simulink model "Current_Controller"  (Simulink 8.9)
settings: Solver=VariableStepAuto  StartTime=0.0  StopTime=0.5  RelTol=1e-3
libraries: simulink x1
settings Model: Creator=MONSTER  LastModifiedBy=MONSTER
settings DataIOCC: LimitDataPoints=off  SaveFormat=Dataset  SignalLoggingSaveFormat=Dataset
settings OptimizationCC: LifeSpan=auto
settings DebuggingCC: UnderspecifiedInitializationDetection=Simplified  MergeDetectMultiDrivingBlocksExec=error  FcnCallInpInsideContextMsg=error  StateNameClashWarn=none  SFUnexpectedBacktrackingDiag=error  SFNoUnconditionalDefaultTransitionDiag=error  SFExecutionAtInitializationDiag=warning
settings HardwareCC: ProdBitPerPointer=64  ProdBitPerSizeT=64  ProdBitPerPtrDiffT=64  ProdLargestAtomicFloat=Float  ProdIntDivRoundTo=Zero  ProdEndianess=LittleEndian  ProdWordSize=64  ProdHWDeviceType=Intel->x86-64 (Windows64)
settings ModelReferenceCC: PropagateSignalLabelsOutOfModel=on
settings GRTTargetCC: TargetLangStandard=C99 (ISO)  GeneratePreprocessorConditionals=Use local settings  CombineOutputUpdateFcns=on  GRTInterface=off
settings ConfigComp: CovMetricSettings=dwe  CovHtmlReporting=off  CovSaveCumulativeToWorkspaceVar=off  CovSaveSingleToWorkspaceVar=off  CovExternalEMLEnable=on

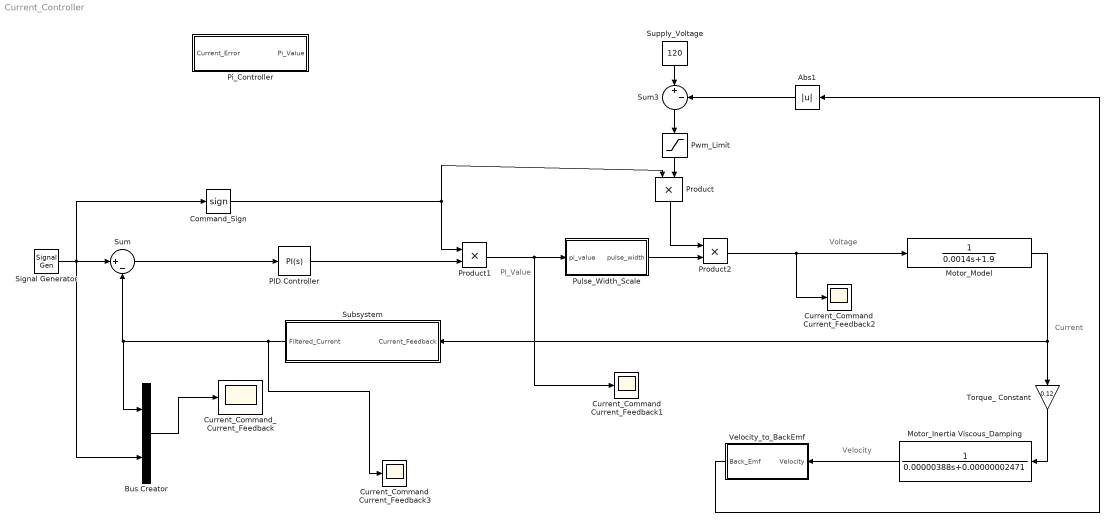
== system Current_Controller ==
  note: Velocity
  note: Current
  note: Voltage
  note: PI_Value
  Abs1 : Abs
  Bus Creator : BusCreator  Inputs=2
  Command_Sign : Signum
  Current_Command Current_Feedback1 : Scope
  Current_Command Current_Feedback2 : Scope
  Current_Command Current_Feedback3 : Scope
  "Current_Command_ Current_Feedback " : Scope
  Motor_Inertia Viscous_Damping : TransferFcn  Denominator=[0.00000388 0.00000002471]
  Motor_Model : TransferFcn  Denominator=[0.0014 1.9]
  PID Controller : simulink/Continuous/PID Controller  Controller=PI  TimeDomain=Continuous-time  SampleTime=-1  IntegratorMethod=Forward Euler  FilterMethod=Forward Euler  Form=Parallel  UseFilter=on  ControllerParametersSource=internal  P=10  I=1000  D=0.1  N=100  InitialConditionSource=internal  InitialConditionForIntegrator=0  InitialConditionForFilter=0  ExternalReset=none  LimitOutput=off  UpperSaturationLimit=inf  LowerSaturationLimit=-inf  LinearizeAsGain=on  AntiWindupMode=none  Kb=1  TrackingMode=off  Kt=1  PParamMin=[]  PParamMax=[]  IParamMin=[]  IParamMax=[]  DParamMin=[]  DParamMax=[]  NParamMin=[]  NParamMax=[]  KbParamMin=[]  KbParamMax=[]  KtParamMin=[]  KtParamMax=[]  POutMin=[]  POutMax=[]  IOutMin=[]  IOutMax=[]  DOutMin=[]  DOutMax=[]  NOutMin=[]  NOutMax=[]  KbOutMin=[]  KbOutMax=[]  KtOutMin=[]  KtOutMax=[]  IntegratorOutMin=[]  IntegratorOutMax=[]  FilterOutMin=[]  FilterOutMax=[]  SumOutMin=[]  SumOutMax=[]  SumI1OutMin=[]  SumI1OutMax=[]  SumI2OutMin=[]  SumI2OutMax=[]  SumI3OutMin=[]  SumI3OutMax=[]  SumDOutMin=[]  SumDOutMax=[]  SaturationOutMin=[]  SaturationOutMax=[]  IntegratorContinuousStateAttributes=''  IntegratorStateMustResolveToSignalObject=off  IntegratorRTWStateStorageClass=Auto  FilterContinuousStateAttributes=''  FilterStateMustResolveToSignalObject=off  FilterRTWStateStorageClass=Auto  DifferentiatorICPrevScaledInput=0  DifferentiatorOutMin=[]  DifferentiatorOutMax=[]  InitialConditionSetting=State (most efficient)
  Pi_Controller : Subsystem
  Product : Product
  Product1 : Product
  Product2 : Product
  Pulse_Width_Scale : Subsystem
  Pwm_Limit : Saturate  UpperLimit=120  LowerLimit=0
  Signal Generator : SignalGenerator  WaveForm=square  Amplitude=10  Frequency=200
  Subsystem : Subsystem
  Sum : Sum  Inputs=|+-
  Sum3 : Sum  Inputs=|+-
  Supply_Voltage : Constant  Value=120
  Torque_ Constant : Gain  Gain=0.12
  Velocity_to_BackEmf : Subsystem
  wires:
  Subsystem/1("Filtered_Current ") -> Current_Command Current_Feedback3/1, Bus Creator/1, Sum/2
  Signal Generator/1 -> Bus Creator/2, Command_Sign/1, Sum/1
  Product1/1 -> Current_Command Current_Feedback1/1, Pulse_Width_Scale/1(pi_value)
  Pulse_Width_Scale/1(pulse_width) -> Product2/2
  Command_Sign/1 -> Product1/1, Product/1
  Torque_ Constant/1 -> Motor_Inertia Viscous_Damping/1
  Motor_Inertia Viscous_Damping/1 -> Velocity_to_BackEmf/1(Velocity)
  PID Controller/1 -> Product1/2
  Motor_Model/1 -> Subsystem/1(Current_Feedback), Torque_ Constant/1
  Product2/1 -> Current_Command Current_Feedback2/1, Motor_Model/1
  Bus Creator/1 -> "Current_Command_ Current_Feedback "/1
  Sum/1 -> PID Controller/1
  Product/1 -> Product2/1
  Sum3/1 -> Pwm_Limit/1
  Supply_Voltage/1 -> Sum3/1
  Velocity_to_BackEmf/1(Back_Emf) -> Abs1/1
  Abs1/1 -> Sum3/2
  Pwm_Limit/1 -> Product/2

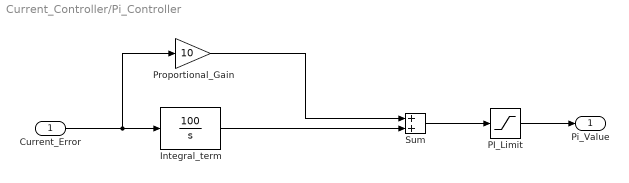
== system Current_Controller/Pi_Controller ==
  "Current_Error " : Inport
  "Integral_term " : TransferFcn  Numerator=100  Denominator=[1 0]
  PI_Limit : Saturate  UpperLimit=1  LowerLimit=-1
  Proportional_Gain : Gain  Gain=10
  Sum : Sum
  "Pi_Value " : Outport
  wires:
  PI_Limit/1 -> "Pi_Value "/1
  Sum/1 -> PI_Limit/1
  Proportional_Gain/1 -> Sum/1
  "Integral_term "/1 -> Sum/2
  "Current_Error "/1 -> Proportional_Gain/1, "Integral_term "/1

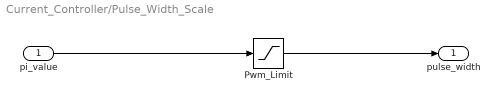
== system Current_Controller/Pulse_Width_Scale ==
  pi_value : Inport
  Pwm_Limit : Saturate  UpperLimit=20  LowerLimit=-20
  pulse_width : Outport
  wires:
  Pwm_Limit/1 -> pulse_width/1
  pi_value/1 -> Pwm_Limit/1

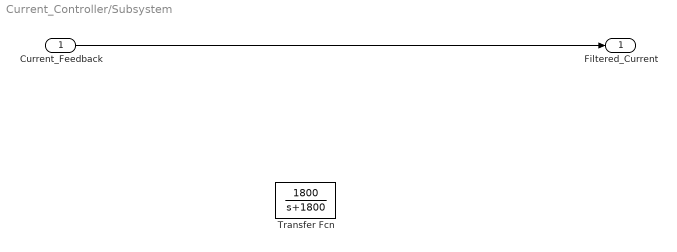
== system Current_Controller/Subsystem ==
  Current_Feedback : Inport
  Transfer Fcn : TransferFcn  Numerator=[1800]  Denominator=[1 1800]
  "Filtered_Current " : Outport
  wires:
  Current_Feedback/1 -> "Filtered_Current "/1

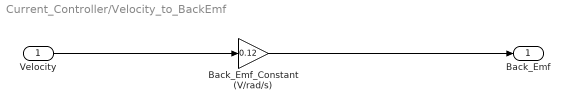
== system Current_Controller/Velocity_to_BackEmf ==
  Velocity : Inport
  Back_Emf_Constant (V/rad/s) : Gain  Gain=0.12
  Back_Emf : Outport
  wires:
  Velocity/1 -> Back_Emf_Constant (V/rad/s)/1
  Back_Emf_Constant (V/rad/s)/1 -> Back_Emf/1
